simulink model "test_slx"  (R2022b)
settings: Solver=VariableStepAuto  StartTime=0.0  StopTime=inf  FixedStep=Ts  RelTol=1e-3
libraries: autolibshared x1
settings Model: PacingRate=0.100000  Creator=DDing  LastModifiedBy=USER
settings DataIOCC: ReturnWorkspaceOutputs=off

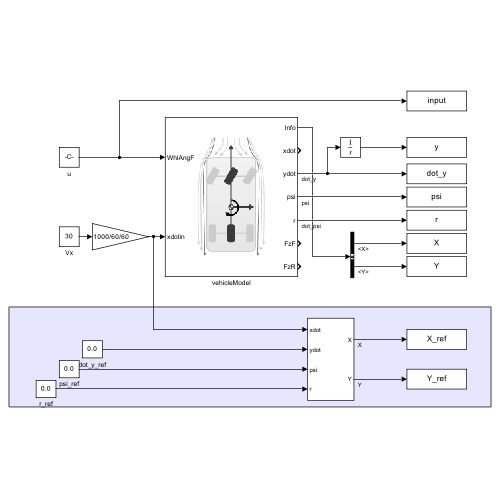
[thumbnail: Simulink's stored preview of the top-level diagram]
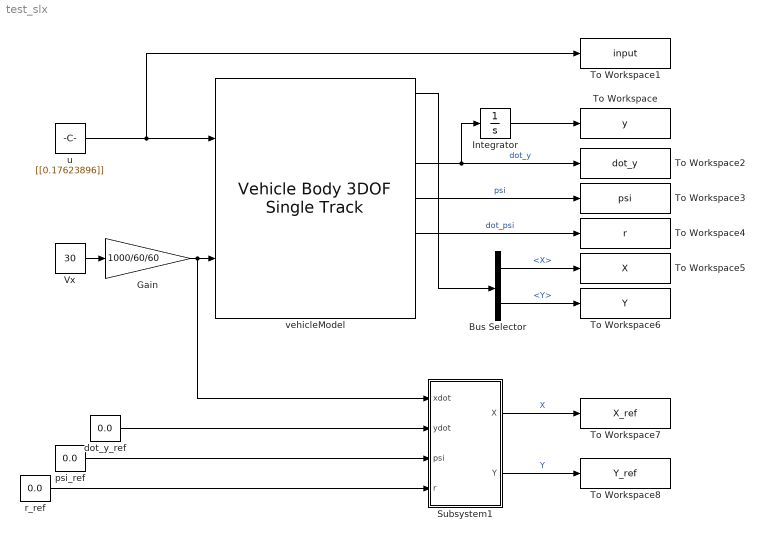
== system test_slx ==
  Bus Selector : BusSelector  OutputSignals=InertFrm.Cg.Disp.X,InertFrm.Cg.Disp.Y
  Gain : Gain  Gain=1000/60/60
  Integrator : Integrator
  Subsystem1 : Subsystem
  To Workspace : ToWorkspace  VariableName=y  SampleTime=-1
      settings: MaxDataPoints=1  Save2DSignal=2-D array (concatenate along first dimension)
  To Workspace1 : ToWorkspace  VariableName=input  SampleTime=-1
      settings: MaxDataPoints=1  Save2DSignal=2-D array (concatenate along first dimension)
  To Workspace2 : ToWorkspace  VariableName=dot_y  SampleTime=-1
      settings: MaxDataPoints=1  Save2DSignal=2-D array (concatenate along first dimension)
  To Workspace3 : ToWorkspace  VariableName=psi  SampleTime=-1
      settings: MaxDataPoints=1  Save2DSignal=2-D array (concatenate along first dimension)
  To Workspace4 : ToWorkspace  VariableName=r  SampleTime=-1
      settings: MaxDataPoints=1  Save2DSignal=2-D array (concatenate along first dimension)
  To Workspace5 : ToWorkspace  VariableName=X  SampleTime=-1
      settings: MaxDataPoints=1  Save2DSignal=2-D array (concatenate along first dimension)
  To Workspace6 : ToWorkspace  VariableName=Y  SampleTime=-1
      settings: MaxDataPoints=1  Save2DSignal=2-D array (concatenate along first dimension)
  To Workspace7 : ToWorkspace  VariableName=X_ref  SampleTime=-1
      settings: MaxDataPoints=1  Save2DSignal=2-D array (concatenate along first dimension)
  To Workspace8 : ToWorkspace  VariableName=Y_ref  SampleTime=-1
      settings: MaxDataPoints=1  Save2DSignal=2-D array (concatenate along first dimension)
  Vx : Constant  Value=30
  dot_y_ref : Constant  Value=0.0
  psi_ref : Constant  Value=0.0
  r_ref : Constant  Value=0.0
  u : Constant  Value=[[0.17623896]]
  vehicleModel : autolibshared/Vehicle Body 3DOF Single Track  trackMode=Single (bicycle)  inputMode=External longitudinal velocity  frontSteerMode=on  rearSteerMode=off  windMode=off  muMode=off  extFMode=off  extMMode=off  htchFMode=off  htchMMode=off  extXo=off  extpsio=off  extxdoto=off  extro=off  extYo=off  extTamb=off  extydoto=off  aMode=2  NF=2  NR=2  m=1573  a=1.1  b=1.58  h=0.35  dh=1  hh=0.2  X_o=[[1.47449177]]  xdot_o=30  CalphaMode=off  sigmaMode=off  d=0  hl=0  w=[1.4,1.4]  Cy_f=80000  Cy_r=80000  sigma_f=.1  sigma_r=.1  alpha_f_brk=[-.1 .1]  Cy_f_data=[-9e3 9e3]  alpha_r_brk=[-.1 .1]  Cy_r_data=[-9e3 9e3]  Y_o=[[-0.04543074]]  ydot_o=[[0.0276248]]  Izz=2873  psi_o=[[0.00363694]]  r_o=[[-0.00722932]]  Af=2  Cd=.3  Cl=.1  Cpm=.1  beta_w=[0 0.01:0.01:0.3]  Cs=[0 0.01:0.01:0.3]  Cym=[0 1e-6:0.01:0.3]  Pabs=101325  Tair=273  g=9.81  mu=1  xdot_tol=.01  Fznom=9.81*1573  Fxtire_sat=7e4  Fytire_sat=7e4  longOff=0  latOff=0  vertOff=0  wrapAng=off
  wires:
  Vx/1 -> Gain/1
  Gain/1 -> Subsystem1/1(xdot), vehicleModel/2
  u/1 -> To Workspace1/1, vehicleModel/1
  vehicleModel/3 -> Integrator/1, To Workspace2/1  "dot_y"
  vehicleModel/4 -> To Workspace3/1  "psi"
  vehicleModel/5 -> To Workspace4/1  "dot_psi"
  Integrator/1 -> To Workspace/1
  vehicleModel/1 -> Bus Selector/1
  Bus Selector/1 -> To Workspace5/1  "<X>"
  Bus Selector/2 -> To Workspace6/1  "<Y>"
  dot_y_ref/1 -> Subsystem1/2(ydot)
  Subsystem1/1(X) -> To Workspace7/1  "X"
  Subsystem1/2(Y) -> To Workspace8/1  "Y"
  psi_ref/1 -> Subsystem1/3(psi)
  r_ref/1 -> Subsystem1/4(r)

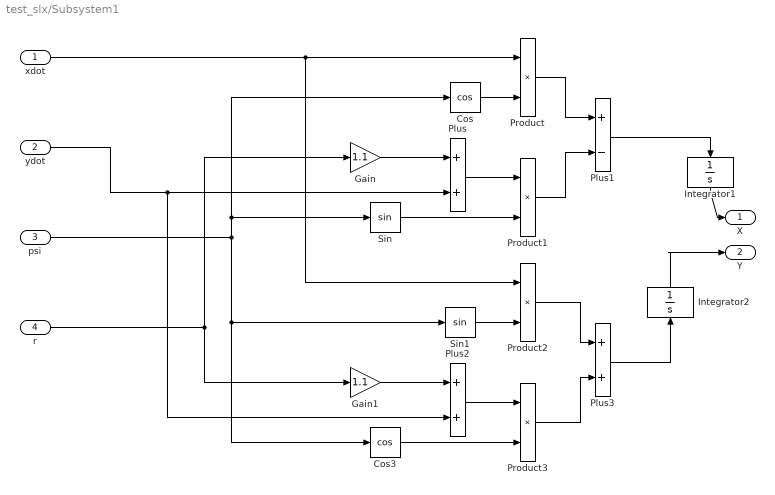
== system test_slx/Subsystem1 ==
  xdot : Inport
  ydot : Inport  Port=2
  psi : Inport  Port=3
  r : Inport  Port=4
  Cos : Trigonometry  Operator=cos
  Cos3 : Trigonometry  Operator=cos
  Gain : Gain  Gain=1.1
  Gain1 : Gain  Gain=1.1
  Integrator1 : Integrator
  Integrator2 : Integrator
  Plus : Sum
  Plus1 : Sum  Inputs=+-
  Plus2 : Sum
  Plus3 : Sum
  Product{,1..3} (4 alike) : Product
  Sin : Trigonometry
  Sin1 : Trigonometry
  X : Outport
  Y : Outport  Port=2
  wires:
  Integrator2/1 -> Y/1
  Integrator1/1 -> X/1
  Product/1 -> Plus1/1
  Plus3/1 -> Integrator2/1
  Gain/1 -> Plus/1
  Cos/1 -> Product/2
  ydot/1 -> Plus2/2, Plus/2
  psi/1 -> Sin/1, Cos/1, Cos3/1, Sin1/1
  Plus2/1 -> Product3/1
  Product2/1 -> Plus3/1
  Cos3/1 -> Product3/2
  Product1/1 -> Plus1/2
  Plus1/1 -> Integrator1/1
  r/1 -> Gain/1, Gain1/1
  Sin/1 -> Product1/2
  Plus/1 -> Product1/1
  xdot/1 -> Product/1, Product2/1
  Gain1/1 -> Plus2/1
  Product3/1 -> Plus3/2
  Sin1/1 -> Product2/2
